simulink model "dataset_simulation"  (R2025b)
settings: Solver=ode23t  StartTime=0.0  StopTime=30  MaxStep=0.0005  RelTol=1e-3
model workspace (MATLAB code in the model file):
  | p = servo_params();
settings Model: Creator=alessandro  LastModifiedBy=alessandro

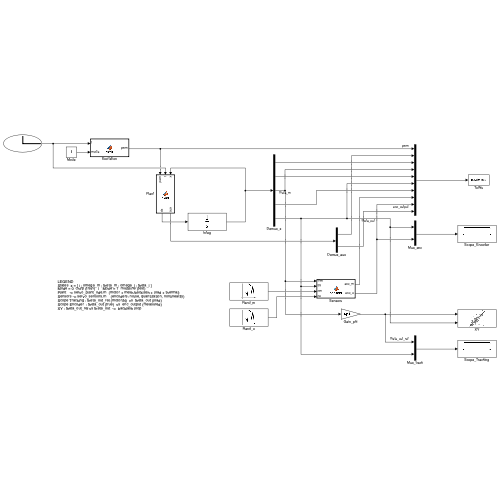
[thumbnail: Simulink's stored preview of the top-level diagram]
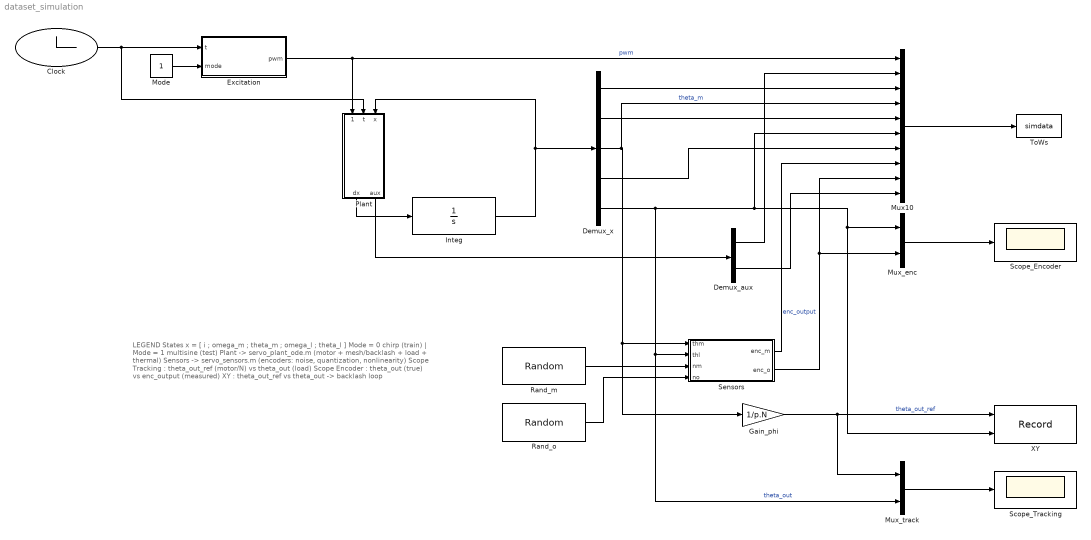
== system dataset_simulation ==
  note: LEGEND
      | States  x = [ i ; omega_m ; theta_m ; omega_l ; theta_l ]
      | Mode = 0  chirp (train)   |   Mode = 1  multisine (test)
      | Plant   -> servo_plant_ode.m  (motor + mesh/backlash + load + thermal)
      | Sensors -> servo_sensors.m    (encoders: noise, quantization, nonlinearity)
      | Scope Tracking : theta_out_ref (motor/N)  vs  theta_out (load)
      | Scope Encoder  : theta_out (true)  vs  enc_output (measured)
      | XY : theta_out_ref vs theta_out  ->  backlash loop
  Clock : Clock
  Demux_aux : Demux  Outputs=2
  Demux_x : Demux  Outputs=5
  Excitation : MATLAB Function  TreatAsAtomicUnit=on
  Gain_phi : Gain  Gain=1/p.N
  Integ : Integrator  InitialCondition=[0;0;0;0;0]
  Mode : Constant
  Mux10 : Mux  Inputs=10
  Mux_enc : Mux  Inputs=2
  Mux_track : Mux  Inputs=2
  Plant : MATLAB Function  TreatAsAtomicUnit=on
  Rand_m : RandomNumber  Variance=p.enc_m_noise^2  Seed=12345  SampleTime=p.dt
  Rand_o : RandomNumber  Variance=p.enc_o_noise^2  Seed=67890  SampleTime=p.dt
  Scope_Encoder : Scope
      settings: ActiveDisplayYMinimum=-0.49403768749841936  ActiveDisplayYMaximum=0.18570754913340543
  Scope_Tracking : Scope
      settings: ActiveDisplayYMinimum=-1  ActiveDisplayYMaximum=1
  Sensors : MATLAB Function  TreatAsAtomicUnit=on
  ToWs : ToWorkspace  VariableName=simdata  SampleTime=-1
  XY : Record  NumPorts=2.0  FileSettingsInternal="{\"entries\":[{\"content\":{\"excelSettings\":{\"content\":{},\"type\":\"Streamout.ExcelSettings\"},\"parquetSettings\":{\"content\":{},\"type\":\"Streamout.ParquetSettings\"}},\"type\":\"Streamout.FileSettingStorage\",\"uuid\":\"\"}],\"packageUris\":[\"http:\\/\\/schema.mathworks.com\\/mf0\\/streamout_blocks\\/R2020a\"],\"version\":\"1.0\"}"  FrameSettings=[0, 0]  Layout=[1 1]  SignalsInternal="{\"entries\":[{\"content\":{\"signals\":[{\"content\":{\"blockPath\":[],\"dimensions\":[1,1],\"domain\":\"\",\"lineColor\":\"#a2142f\",\"plots\":[ 1 ],\"port\":1,\"sid\":[\"\"],\"signalID\":1,\"signalName\":\"theta_out_ref\"},\"type\":\"RecordBlkView.Signal\",\"uuid\":\"\"},{\"content\":{\"blockPath\":[],\"dimensions\":[1,1],\"domain\":\"\",\"lineColor\":\"#139fff\",\"plots\":[ 1 ],\"port\":2,\"sid\":[\"\"],\"signalID\":2,\"signalName\":\"theta_out\"},\"type\":\"RecordBlkView.Signal\",\"uuid\":\"\"}]},\"type\":\"RecordBlkView.InputSignals\",\"uuid\":\"\"}],\"packageUris\":[\"http:\\/\\/schema.mathworks.com\\/mf0\\/streamout_blocks\\/R2020a\"],\"version\":\"1.0\"}"  VisualizationBindings="{\"xyplotplugin\":{\"info\":[{\"series\":[{\"bindingParametersList\":[{\"parameter\":\"X-Axis\",\"signalID\":1,\"signalName\":\"theta_out_ref\"},{\"parameter\":\"Y-Axis\",\"signalID\":2,\"signalName\":\"theta_out\"}],\"seriesID\":0}],\"subplotID\":1}]}}"  CompatibilityTag=XY
  wires:
  Mux_track/1 -> Scope_Tracking/1
  Sensors/2(enc_o) -> Mux10/9, Mux_enc/2  "enc_output"
  Rand_o/1 -> Sensors/4(no)
  Demux_aux/2 -> Mux10/10
  Rand_m/1 -> Sensors/3(nm)
  Clock/1 -> Plant/2(t), Excitation/1(t)
  Demux_x/4 -> Mux10/7
  Demux_x/1 -> Mux10/3
  Mux_enc/1 -> Scope_Encoder/1
  Integ/1 -> Demux_x/1, Plant/3(x)
  Mux10/1 -> ToWs/1
  Demux_x/5 -> Sensors/2(thl), Mux_track/2, XY/2, Mux_enc/1, Mux10/6  "theta_out"
  Mode/1 -> Excitation/2(mode)
  Sensors/1(enc_m) -> Mux10/8
  Plant/1(dx) -> Integ/1
  Demux_aux/1 -> Mux10/2
  Demux_x/3 -> Gain_phi/1, Sensors/1(thm), Mux10/4  "theta_m"
  Demux_x/2 -> Mux10/5
  Excitation/1(pwm) -> Plant/1(pwm), Mux10/1  "pwm"
  Gain_phi/1 -> Mux_track/1, XY/1  "theta_out_ref"
  Plant/2(aux) -> Demux_aux/1

== matlab function dataset_simulation/Plant ==
  data: pwm input; dx output; t input; x input; aux output
function [dx, aux] = plant(pwm, t, x)
    [dx, aux] = servo_plant_ode(pwm, t, x);
end

== matlab function dataset_simulation/Excitation ==
  data: t input; pwm output; mode input
function pwm = excit(t, mode)
    pwm = servo_excitation(t, mode);
end

== matlab function dataset_simulation/Sensors ==
  data: thm input; enc_m output; thl input; nm input; no input; enc_o output
function [enc_m, enc_o] = sensors(thm, thl, nm, no)
    [enc_m, enc_o] = servo_sensors(thm, thl, nm, no);
end
